simulink model "VibrationIsolation"  (R2020b)
settings: Solver=FixedStepAuto  StartTime=0.0  StopTime=T  FixedStep=Ts  RelTol=1e-3
values from neighbouring files (symbols this model uses):
  ainFlag = 1    [Sim01_OpenLoop.m]    (also in Sim02_ClosedLoop.m = 3)
  Kd = 0    [Sim02_ClosedLoop.m]
  Ki = 200    [Sim02_ClosedLoop.m]
  Kp = 150    [Sim02_ClosedLoop.m]
  N = 100    [Sim02_ClosedLoop.m]
  omg2 = omega^2    (= 3947.84176044)    [Sim01_OpenLoop.m]    (also in Sim02_ClosedLoop.m = 467.928899623)
  Ts = 1e-3    (= 0.001)    [Sim01_OpenLoop.m]    (also in Sim02_ClosedLoop.m)
  v0 = 0    [Sim01_OpenLoop.m]    (also in Sim02_ClosedLoop.m)
  x0 = 0    [Sim01_OpenLoop.m]    (also in Sim02_ClosedLoop.m)
  xi = 2*omega*0.3    (= 37.6991118431)    [Sim01_OpenLoop.m]    (also in Sim02_ClosedLoop.m)
libraries: cstblocks x2, pid_lib x1, simulink x1
settings Model: Creator=xiaocy  LastModifiedBy=xiaocy
settings DataIOCC: SaveOutput=off  SignalLogging=off  DSMLogging=off  SaveTime=off  ReturnWorkspaceOutputs=off

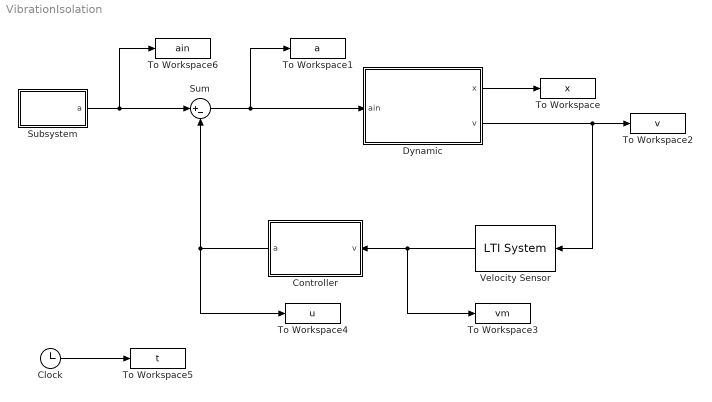
== system VibrationIsolation ==
  Clock : Clock
  Controller : Subsystem  Variant=on
  Dynamic : Subsystem
      mask Display: disp('2nd System')
  Subsystem : Subsystem
      mask Display: disp('Acceleration')
  Sum : Sum  Inputs=|+-
  To Workspace : ToWorkspace  VariableName=x  SampleTime=Ts
  To Workspace1 : ToWorkspace  VariableName=a  SampleTime=Ts
  To Workspace2 : ToWorkspace  VariableName=v  SampleTime=Ts
  To Workspace3 : ToWorkspace  VariableName=vm  SampleTime=Ts
  To Workspace4 : ToWorkspace  VariableName=u  SampleTime=Ts
  To Workspace5 : ToWorkspace  VariableName=t  SampleTime=Ts
  To Workspace6 : ToWorkspace  VariableName=ain  SampleTime=Ts
  Velocity Sensor : cstblocks/LTI System  sys=Hs  IC=[]
  wires:
  Subsystem/1(a) -> To Workspace6/1, Sum/1
  Controller/1(a) -> To Workspace4/1, Sum/2
  Dynamic/1(x) -> To Workspace/1
  Sum/1 -> To Workspace1/1, Dynamic/1(ain)
  Clock/1 -> To Workspace5/1
  Dynamic/2(v) -> Velocity Sensor/1, To Workspace2/1
  Velocity Sensor/1 -> To Workspace3/1, Controller/1(v)

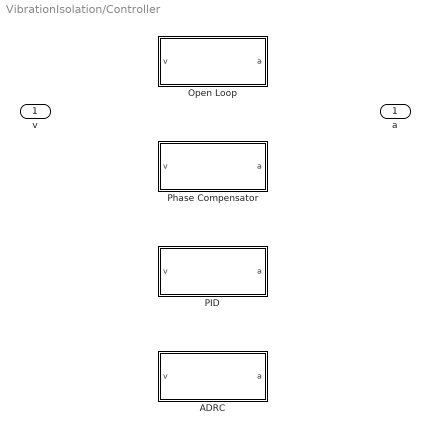
== system VibrationIsolation/Controller ==
  v : Inport
  ADRC : Subsystem  VariantControl=ctrlFlag == 3
  Open Loop : Subsystem  VariantControl=ctrlFlag == 0
  PID : Subsystem  VariantControl=ctrlFlag == 2
  Phase Compensator : Subsystem  VariantControl=ctrlFlag == 1
  a : Outport

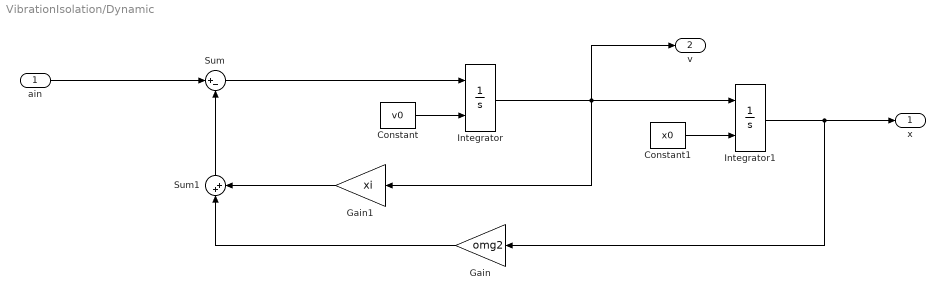
== system VibrationIsolation/Dynamic ==
  ain : Inport
  Constant : Constant  Value=v0
  Constant1 : Constant  Value=x0
  Gain : Gain  Gain=omg2
  Gain1 : Gain  Gain=xi
  Integrator : Integrator  InitialConditionSource=external
  Integrator1 : Integrator  InitialConditionSource=external
  Sum : Sum  Inputs=|+-
  Sum1 : Sum  Inputs=|++
  x : Outport
  v : Outport  Port=2
  wires:
  ain/1 -> Sum/1
  Integrator/1 -> v/1, Gain1/1, Integrator1/1
  Constant/1 -> Integrator/2
  Constant1/1 -> Integrator1/2
  Sum/1 -> Integrator/1
  Integrator1/1 -> x/1, Gain/1
  Sum1/1 -> Sum/2
  Gain/1 -> Sum1/1
  Gain1/1 -> Sum1/2

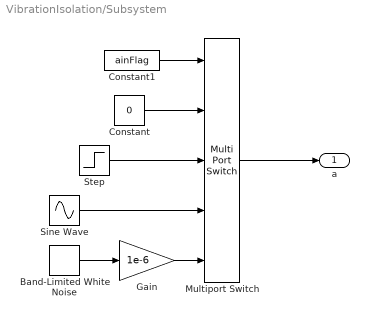
== system VibrationIsolation/Subsystem ==
  Band-Limited White Noise : simulink/Sources/Band-Limited White Noise  Cov=1/2  Ts=Ts  seed=18468
  Constant : Constant  Value=0
  Constant1 : Constant  Value=ainFlag
  Gain : Gain  Gain=1e-6
  Multiport Switch : MultiPortSwitch  DataPortOrder=Zero-based contiguous  Inputs=4  zeroidx=on
  Sine Wave : Sin  Amplitude=1e-6  Frequency=0.1*2*pi  SampleTime=0
  Step : Step  Time=0  After=1e-6  SampleTime=0
  a : Outport
  wires:
  Multiport Switch/1 -> a/1
  Step/1 -> Multiport Switch/3
  Constant/1 -> Multiport Switch/2
  Constant1/1 -> Multiport Switch/1
  Sine Wave/1 -> Multiport Switch/4
  Gain/1 -> Multiport Switch/5
  Band-Limited White Noise/1 -> Gain/1

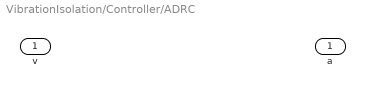
== system VibrationIsolation/Controller/ADRC ==
  v : Inport
  a : Outport

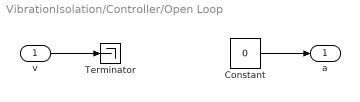
== system VibrationIsolation/Controller/Open Loop ==
  v : Inport
  Constant : Constant  Value=0
  Terminator : Terminator
  a : Outport
  wires:
  v/1 -> Terminator/1
  Constant/1 -> a/1

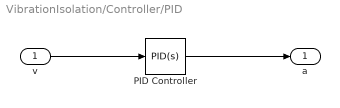
== system VibrationIsolation/Controller/PID ==
  v : Inport
  PID Controller : pid_lib/PID Controller  Controller=PID  Form=Ideal  TimeDomain=Continuous-time  UseExternalTs=off  SampleTime=-1  IntegratorMethod=Forward Euler  FilterMethod=Forward Euler  ControllerParametersSource=internal  P=Kp  I=Ki  D=Kd  UseFilter=on  N=N  TunerSelectOption=Transfer Function Based (PID Tuner App)  InitialConditionSource=internal  InitialConditionForIntegrator=0  InitialConditionForFilter=0  DifferentiatorICPrevScaledInput=0  ExternalReset=none  TrackingMode=off  Kt=1  LimitOutput=off  SatLimitsSource=internal  UpperSaturationLimit=inf  LowerSaturationLimit=-inf  LinearizeAsGain=on  AntiWindupMode=none  Kb=1  POutMin=[]  POutMax=[]  IOutMin=[]  IOutMax=[]  DOutMin=[]  DOutMax=[]  NOutMin=[]  NOutMax=[]  SumOutMin=[]  SumOutMax=[]  SaturationOutMin=[]  SaturationOutMax=[]  PParamMin=[]  PParamMax=[]  IParamMin=[]  IParamMax=[]  DParamMin=[]  DParamMax=[]  NParamMin=[]  NParamMax=[]  KbParamMin=[]  KbParamMax=[]  KtParamMin=[]  KtParamMax=[]  KbOutMin=[]  KbOutMax=[]  KtOutMin=[]  KtOutMax=[]  IntegratorOutMin=[]  IntegratorOutMax=[]  FilterOutMin=[]  FilterOutMax=[]  SumI1OutMin=[]  SumI1OutMax=[]  SumI2OutMin=[]  SumI2OutMax=[]  SumI3OutMin=[]  SumI3OutMax=[]  SumI4OutMin=[]  SumI4OutMax=[]  SumDOutMin=[]  SumDOutMax=[]  DifferentiatorOutMin=[]  DifferentiatorOutMax=[]  FilterDiffOutCoefMin=[]  FilterDiffOutCoefMax=[]  ReciprocalOutMin=[]  ReciprocalOutMax=[]  SumDenOutMin=[]  SumDenOutMax=[]  SumNumOutMin=[]  SumNumOutMax=[]  DivideOutMin=[]  DivideOutMax=[]  UdiffTsProdOutMin=[]  UdiffTsProdOutMax=[]  NTsProdOutMin=[]  NTsProdOutMax=[]  UintegralTsProdOutMin=[]  UintegralTsProdOutMax=[]  UngainTsProdOutMin=[]  UngainTsProdOutMax=[]  IntegratorContinuousStateAttributes=''  IntegratorStateMustResolveToSignalObject=off  IntegratorRTWStateStorageClass=Auto  FilterContinuousStateAttributes=''  FilterStateMustResolveToSignalObject=off  FilterRTWStateStorageClass=Auto  ParallelPVariant=Passthrough  IdealPVariant=InternalParameters  IVariant=InternalParameters  DVariant=InternalParameters  IntegratorVariant=Continuous  SatVariant=Disabled  AWVariant=Passthrough  PCopyVariant=Disabled  TRVariant=Disabled  FdbkBlocksVariant=Forward  IdealPFdbkVariant=Disabled  SatFdbkVariant=Disabled  DerivativeFilterVariant=ContFilter  NVariant=InternalParameters  NCopyVariant=Disabled  FilterICVariant=InternalICsFilter  IntegratorICVariant=InternalICs  ExternalResetVariant=Disabled  TRSumVariant=Passthrough  SumFdbkVariant=Disabled  SumVariant=Sum_PID  TsampFilterVariant=InternalTs  TsampNgainVariant=Passthrough  TsampIntegralVariant=Passthrough  ExternalSaturationOutDataTypeStr=Inherit: Same as second input
  a : Outport
  wires:
  v/1 -> PID Controller/1
  PID Controller/1 -> a/1

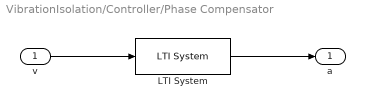
== system VibrationIsolation/Controller/Phase Compensator ==
  v : Inport
  LTI System : cstblocks/LTI System  sys=Hpc  IC=[]
  a : Outport
  wires:
  v/1 -> LTI System/1
  LTI System/1 -> a/1
